simulink model "test_edge_detect"  (Simulink 6.2)
settings: Solver=ode45  StartTime=0.0  StopTime=35  RelTol=1e-3
libraries: xbsIndex_r3 x4, simulink x1, newfft_library x1
settings Model: LastModifiedBy=mdexter
settings DebuggingCC: SolverPrmCheckMsg=warning

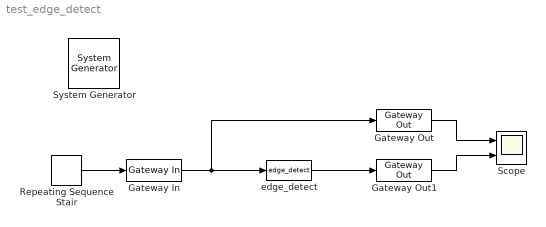
== system test_edge_detect ==
  " System Generator" : xbsIndex_r3/ System Generator  Tag=genX  xilinxfamily=Virtex2  part=xc2v1000  speed=-4  package=bg575  synthesis_tool=XST  directory=./netlist  testbench=off  simulink_period=1  sysclk_period=100  incr_netlist=off  trim_vbits=Everywhere in SubSystem  dbl_ovrd=According to Block Masks  core_generation=According to Block Masks  run_coregen=off  deprecated_control=off  eval_field=0
      settings: AttributesFormatString=System\nGenerator
  Gateway In : xbsIndex_r3/Gateway In  arith_type="Signed  (2's comp)"  n_bits=8  bin_pt=6  quantization=Truncate  overflow=Wrap  period=1  timing_constraint=None  locs_specified=off  LOCs={}  needs_fixed_name=off  dbl_ovrd=off  show_param=off
      settings: xl_area=[0, 0, 0, 0, 0, 0, 0]
  Gateway Out : xbsIndex_r3/Gateway Out  output_type=Double  nbits=8  bin_pt=6  arith_type=Boolean  quantization=Truncate  overflow=Wrap  hdl_port=on  timing_constraint=None  locs_specified=off  LOCs={}  needs_fixed_name=off  show_param=off
      settings: xl_area=[0, 0, 0, 0, 0, 0, 0]
  Gateway Out1 : xbsIndex_r3/Gateway Out  output_type=Double  nbits=8  bin_pt=6  arith_type=Boolean  quantization=Truncate  overflow=Wrap  hdl_port=on  timing_constraint=None  locs_specified=off  LOCs={}  needs_fixed_name=off  show_param=off
      settings: xl_area=[0, 0, 0, 0, 0, 0, 0]
  Repeating Sequence Stair : simulink/Sources/Repeating Sequence Stair  OutValues=[zeros(1,5) ones(1,5) zeros(1,5) 1 0 1 0 1]  tsamp=-1  OutputDataTypeScalingMode=Specify via dialog  OutDataType=float('double')  ConRadixGroup=Best Precision: Vector-wise  OutScaling=2^-12
  Scope : Scope  NumInputPorts=2
      settings: YMin=-5~-5  YMax=5~5
  edge_detect : newfft_library/Utility/edge_detect  edge=Falling  polarity=Active High  xin=floor([0.5:0.5:5])*0.08  yin={[-1,-1,1,1,1,1,1,1,1,1],[1,1,-1,-1,-1,-1,-1,-1,-1,-1],[-1,-1,1,1,1,1,-1,-1,-1,-1]}  xout=1-floor([5:-0.5:0.5])*0.08  yout={[-1,-1,1,1,-1,-1,-1,-1,-1,-1],[-1,-1,1,1,-1,-1,-1,-1,-1,-1],[-1,-1,1,1,-1,-1,1,1,-1,-1]}
      settings: AttributesFormatString=|
      | falling edge
      | active high
  wires:
  Repeating Sequence Stair/1 -> Gateway In/1
  Gateway In/1 -> Gateway Out/1, edge_detect/1
  edge_detect/1 -> Gateway Out1/1
  Gateway Out/1 -> Scope/1
  Gateway Out1/1 -> Scope/2
